simulink model "Simulink_ZT"  (R2019a)
settings: Solver=VariableStepAuto  StartTime=0.0  StopTime=10.0  RelTol=1e-3
values from neighbouring files (symbols this model uses):
  A = [ A11 A12 A13 A14 ... (first row only)    [Praktikum_1.m]    (also in calcZRM.m)
  bv = [B1 ... (first row only)    [Praktikum_1.m]    (also in calcZRM.m)
  cT = [1 0 0 0]    [Praktikum_1.m]    (also in calcZRM.m)
  d = 0    [Praktikum_1.m]    (also in calcZRM.m)
  x0 = [0 0 0 0]    [Praktikum.m]    (also in Praktikum_1.m = [5 0 0 0])
settings Model: Creator=Origilon  LastModifiedBy=Origilon

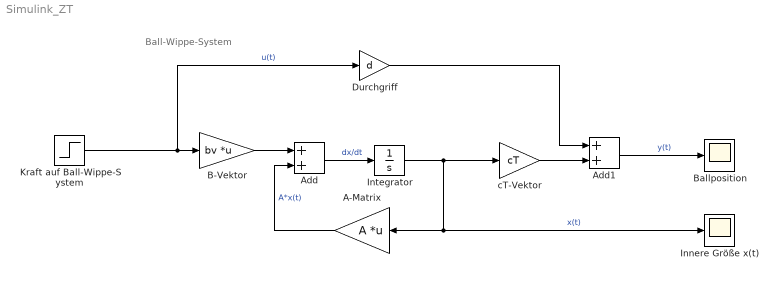
== system Simulink_ZT ==
  note: Ball-Wippe-System
  A-Matrix : Gain  Gain=A  Multiplication=Matrix(K*u) (u vector)
  Add : Sum
  Add1 : Sum
  B-Vektor : Gain  Gain=bv  Multiplication=Matrix(K*u) (u vector)
  "Ballposition " : Scope
  Durchgriff : Gain  Gain=d
  Innere Größe x(t) : Scope
  Integrator : Integrator  InitialCondition=x0
  Kraft auf Ball-Wippe-System : Step  SampleTime=0
  cT-Vektor : Gain  Gain=cT
  wires:
  Kraft auf Ball-Wippe-System/1 -> Durchgriff/1, B-Vektor/1  "u(t)"
  B-Vektor/1 -> Add/1
  Add/1 -> Integrator/1  "dx/dt"
  Integrator/1 -> Innere Größe x(t)/1, A-Matrix/1, cT-Vektor/1  "x(t)"
  cT-Vektor/1 -> Add1/2
  Durchgriff/1 -> Add1/1
  A-Matrix/1 -> Add/2  "A*x(t)"
  Add1/1 -> "Ballposition "/1  "y(t)"
